simulink model "ex5"  (R2020a)
settings: Solver=VariableStepAuto  StartTime=0.0  StopTime=10.0  RelTol=1e-3
libraries: simulink x2

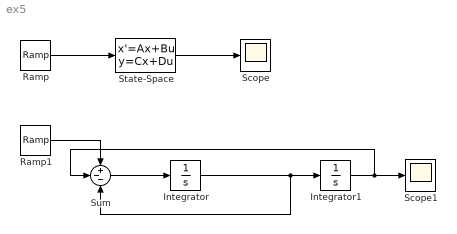
== system ex5 ==
  Integrator : Integrator
  Integrator1 : Integrator
  Ramp : simulink/Sources/Ramp  slope=1  start=0  InitialOutput=0
  Ramp1 : simulink/Sources/Ramp  slope=1  start=0  InitialOutput=0
  Scope : Scope
  Scope1 : Scope
  State-Space : StateSpace  A=[0 1;-1 -1]  B=[0;1]  C=[1 0]  D=[0]  InitialCondition=0
  Sum : Sum  Inputs=+--
  wires:
  Ramp/1 -> State-Space/1
  State-Space/1 -> Scope/1
  Ramp1/1 -> Sum/1
  Sum/1 -> Integrator/1
  Integrator/1 -> Sum/3, Integrator1/1
  Integrator1/1 -> Scope1/1, Sum/2
